simulink model "graz_bci_model"  (R2016a)
settings: Solver=FixedStepDiscrete  StartTime=0.0  StopTime=inf  FixedStep=1/128  RelTol=1e-3
PreLoadFcn:
  | preloadscript
InitFcn:
  | initscript
undefined symbols (not defined in the file): BCI
settings Model: Creator=ABC  LastModifiedBy=christian
settings DataIOCC: LimitDataPoints=on  SaveFormat=Array
settings OptimizationCC: ExpressionDepthLimit=2147483647
settings DebuggingCC: UnderspecifiedInitializationDetection=Classic  MergeDetectMultiDrivingBlocksExec=none  SolverPrmCheckMsg=warning  StateNameClashWarn=warning
settings HardwareCC: ProdBitPerPointer=32  ProdLargestAtomicFloat=None  ProdIntDivRoundTo=Undefined  ProdEndianess=Unspecified  ProdWordSize=32  ProdHWDeviceType=32-bit Generic
settings ModelReferenceCC: UpdateModelReferenceTargets=IfOutOfDate  PropagateSignalLabelsOutOfModel=off
settings SFSimCC: SFSimEcho=off

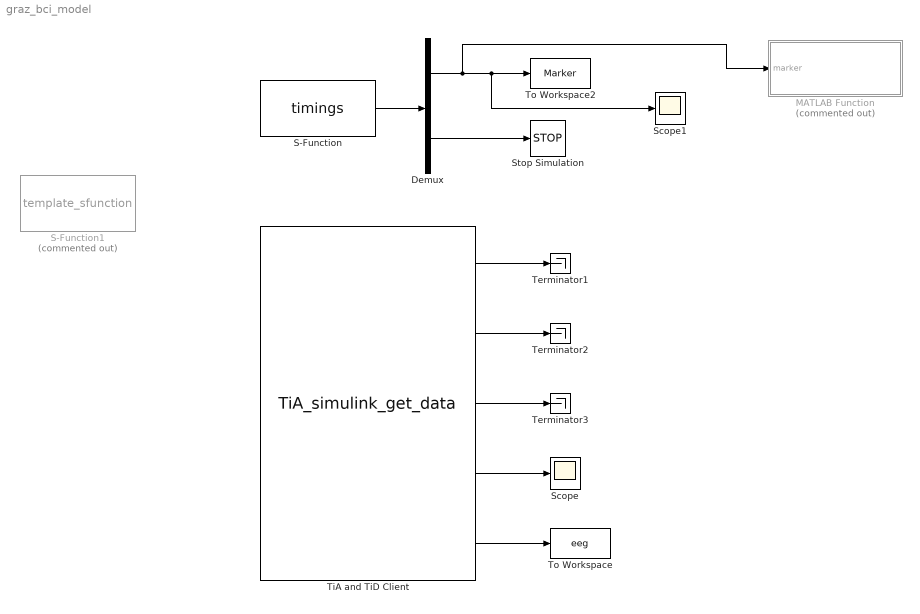
== system graz_bci_model ==
  Demux : Demux  Outputs=2
  MATLAB Function : MATLAB Function  Commented=on  TreatAsAtomicUnit=on
  S-Function : S-Function  FunctionName=timings  SFunctionDeploymentMode=off  EnableBusSupport=off
      mask Display:
      | disp('Timings');
      | port_label('output', 1, 'flags' );
  S-Function1 : S-Function  Commented=on  FunctionName=template_sfunction  SFunctionDeploymentMode=off  EnableBusSupport=off
      mask Display:
      | disp('Timings');
      | port_label('output', 1, 'flags' );
  Scope : Scope
  Scope1 : Scope
  Stop Simulation : Stop
  Terminator1 : Terminator
  Terminator2 : Terminator
  Terminator3 : Terminator
  TiA and TiD Client : S-Function  Priority=1  FunctionName=TiA_simulink_get_data  Parameters=master_fs, master_bs, sig_info , ip, port, proto, tia_version, use_tid, tid_ip, tid_port  SFunctionDeploymentMode=off  EnableBusSupport=off  mask{master_fs=BCI.SampleRate, master_bs=BCI.Blocksize, sig_info=BCI.sig_info, ip=BCI.TiATiD_client.TiA_server_ip, port=BCI.TiATiD_client.TiA_server_port, proto=BCI.TiATiD_client.protocol, tia_version=BCI.TiATiD_client.TiA_version, use_tid=BCI.TiATiD_client.use_TiD, tid_ip=BCI.TiATiD_client.TiD_server_ip, tid_port=BCI.TiATiD_client.TiD_server_port}
      mask prompts: master_fs "TiA server sampe rate"; master_bs "TiA server block size"; sig_info "Signal info structure"; ip "TiA server ip address"; port "TiA server port"; proto "TiA server protocol type"; tia_version "TiA server protocol version"; use_tid "Use TiD Client"; tid_ip "TiD server ip address"; tid_port "TiD server port"
      mask help:
      | This is a combined client to receive raw data via TiA and events via TiD.
      | The packet ID is a unique ascending value for incomming data packets.
      | The timestamp represents the TiA timestamp, which is a uint64 in microseconds
      | since the TiA server start.
      | TiD events are aligned according to the Packet ID
      |
      | The Sys/Sim time port shows the difference between the system time and the
      | simulation time. An ascending value indicates, that the simulation is running
      | too slow! (a slowly decreasing sys/sim time can occur because of rounding
      | errors within the calculation)
      mask Display:
      | global BCI;
      | 
      | disp('TiA/TiD Client');
      | 
      | port_label('output', 1, 'TiD Events' );
      | port_label('output', 2, 'Packet ID' );
      | port_label('output', 3, 'Timestamp' );
      | port_label('output', 4, 'Sys/Sim Time' );
      | 
      | for n = 1:size(BCI.sig_info_labeled,1)
      |   port_label('output', 4+n, num2str(cell2mat(BCI.sig_info_labeled(n,2))) );
      | end
  To Workspace : ToWorkspace  VariableName=eeg  SaveFormat=Timeseries  SampleTime=-1
  To Workspace2 : ToWorkspace  VariableName=Marker  SaveFormat=Timeseries  SampleTime=-1
  wires:
  TiA and TiD Client/4 -> Scope/1
  TiA and TiD Client/1 -> Terminator1/1
  TiA and TiD Client/2 -> Terminator2/1
  TiA and TiD Client/3 -> Terminator3/1
  S-Function/1 -> Demux/1
  Demux/2 -> Stop Simulation/1
  Demux/1 -> MATLAB Function/1(marker), To Workspace2/1, Scope1/1
  TiA and TiD Client/5 -> To Workspace/1

== matlab function graz_bci_model/MATLAB Function ==
  data: marker input
function showParadigm(marker)
%#codegen
switch marker
    
    case 1
        fig = figure('units','normalized','outerposition',[0 0 1 1]);
    case 2 
        set(gcf, 'color', 'b')
    case 3
        set(gcf, 'color', 'g')
    case 4
        set(gcf, 'color', 'w')
    case 5
        set(gcf, 'color', 'b')
end
        
    
    
end
